simulink model "TP2_tanque_simulink_resp_impul"  (R2019b)
settings: Solver=VariableStepAuto  StartTime=0.0  StopTime=1500.0  RelTol=1e-3
values from neighbouring files (symbols this model uses):
  Ad = Hld_zoh.A    [TP2_rutina_minimos_cuadrados.m]    (also in tanque_simulink_param.m)
  alt_tank = 1    [TP2_rutina_minimos_cuadrados.m]    (also in tanque_simulink_param.m)
  ang = pi/3    (= 1.0471975512)    [TP2_rutina_minimos_cuadrados.m]    (also in tanque_simulink_param.m)
  Bd = Hld_zoh.B    [TP2_rutina_minimos_cuadrados.m]    (also in tanque_simulink_param.m)
  Cd = Hld_zoh.C    [TP2_rutina_minimos_cuadrados.m]    (also in tanque_simulink_param.m)
  d_p_apertura = 0.05    [TP2_rutina_minimos_cuadrados.m]    (also in tanque_simulink_param.m)
  Dd = Hld_zoh.D    [TP2_rutina_minimos_cuadrados.m]    (also in tanque_simulink_param.m)
  g = 9.8    [TP2_rutina_minimos_cuadrados.m]    (also in tanque_simulink_param.m)
  h0 = h0_array(i)    [TP2_rutina_minimos_cuadrados.m]    (also in tanque_simulink_param.m)
  p_apertura_lin = Q_ent/(pi*r_apertura^2) / (sqrt(2*g*h0))    [obtener_modelo_lineal.m]
  Q_ent = 0.0035    [TP2_rutina_minimos_cuadrados.m]    (also in tanque_simulink_param.m)
  r_apertura = 0.0254    [TP2_rutina_minimos_cuadrados.m]    (also in tanque_simulink_param.m)
  rad_menor = 0.05    [TP2_rutina_minimos_cuadrados.m]    (also in tanque_simulink_param.m)
  T0 = Ts    (= 1)    [TP2_rutina_minimos_cuadrados.m]    (also in tanque_simulink_param.m)
  Ts = 1    [TP2_rutina_minimos_cuadrados.m]    (also in tanque_simulink_param.m)
settings Model: Creator=Franco  LastModifiedBy=Franco

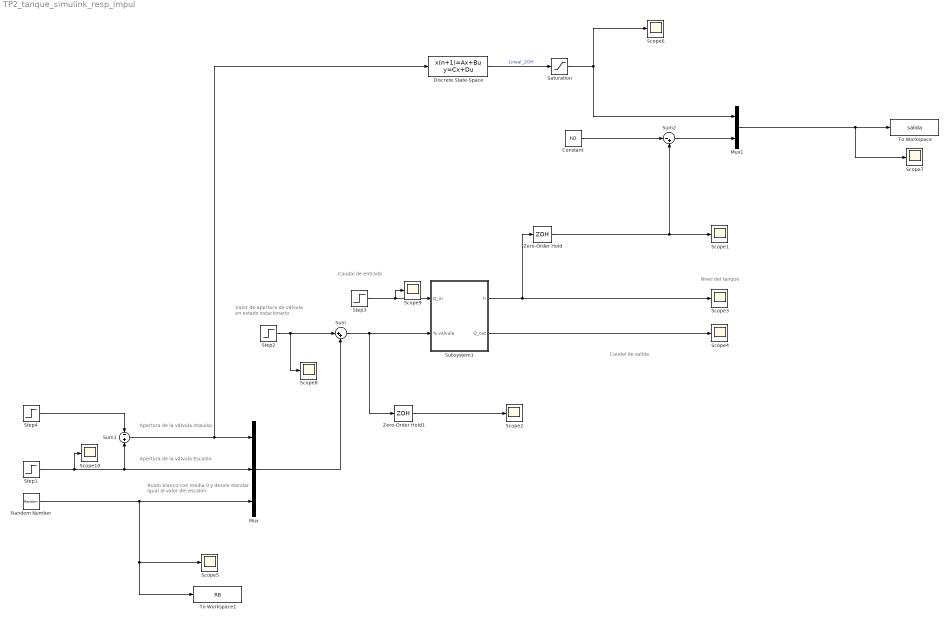
== system TP2_tanque_simulink_resp_impul ==
  note: Ruido blanco con media 0 y
      | desvío standar igual al valor del escalon
  note: Valor de apertura de válvula
      | en estado estacionario
  note: Apertura de la válvula
      | Escalón
  note: Caudal de salida
  note: Nivel del tanque
  note: Apertura de la válvula
      | Impulso
  note: Caudal de entrada
  Constant : Constant  Value=h0
  Discrete State-Space : DiscreteStateSpace  A=Ad  B=Bd  C=Cd  D=Dd  SampleTime=Ts
  Mux : Mux  Inputs=3
  Mux1 : Mux  Inputs=2
  Random Number : RandomNumber  Variance=(p_apertura_lin*d_p_apertura)^2  SampleTime=T0
  Saturation : Saturate  UpperLimit=alt_tank - h0  LowerLimit=-h0
  Scope{1..10} (10 alike) : Scope
  Step1 : Step  Time=T0  After=p_apertura_lin*d_p_apertura  SampleTime=0
  Step2 : Step  Time=T0/100  After=p_apertura_lin  SampleTime=0
  Step3 : Step  Time=T0/100  After=Q_ent  SampleTime=0
  Step4 : Step  Time=T0 + Ts  After=p_apertura_lin*d_p_apertura  SampleTime=0
  Subsystem1 : Subsystem
  Sum : Sum  Inputs=|++
  Sum1 : Sum  Inputs=-+
  Sum2 : Sum  Inputs=|-+
  To Workspace : ToWorkspace  VariableName=salida  SaveFormat=Timeseries  SampleTime=-1
      settings: Save2DSignal=2-D array (concatenate along first dimension)
  To Workspace1 : ToWorkspace  VariableName=RB  SaveFormat=Timeseries  SampleTime=-1
  Zero-Order Hold : ZeroOrderHold
  Zero-Order Hold1 : ZeroOrderHold
  wires:
  Step3/1 -> Scope9/1, Subsystem1/1(Q_in)
  Subsystem1/2(Q_out) -> Scope4/1
  Subsystem1/1(h) -> Zero-Order Hold/1, Scope3/1
  Zero-Order Hold/1 -> Sum2/2, Scope1/1
  Step1/1 -> Scope10/1, Mux/2, Sum1/2
  Zero-Order Hold1/1 -> Scope2/1
  Sum/1 -> Zero-Order Hold1/1, Subsystem1/2(" % válvula")
  Step2/1 -> Scope8/1, Sum/1
  Step4/1 -> Sum1/1
  Mux/1 -> Sum/2
  Random Number/1 -> To Workspace1/1, Scope5/1, Mux/3
  Discrete State-Space/1 -> Saturation/1  "Lineal_ZOH"
  Constant/1 -> Sum2/1
  Sum2/1 -> Mux1/2
  Sum1/1 -> Discrete State-Space/1, Mux/1
  Saturation/1 -> Scope6/1, Mux1/1
  Mux1/1 -> Scope7/1, To Workspace/1

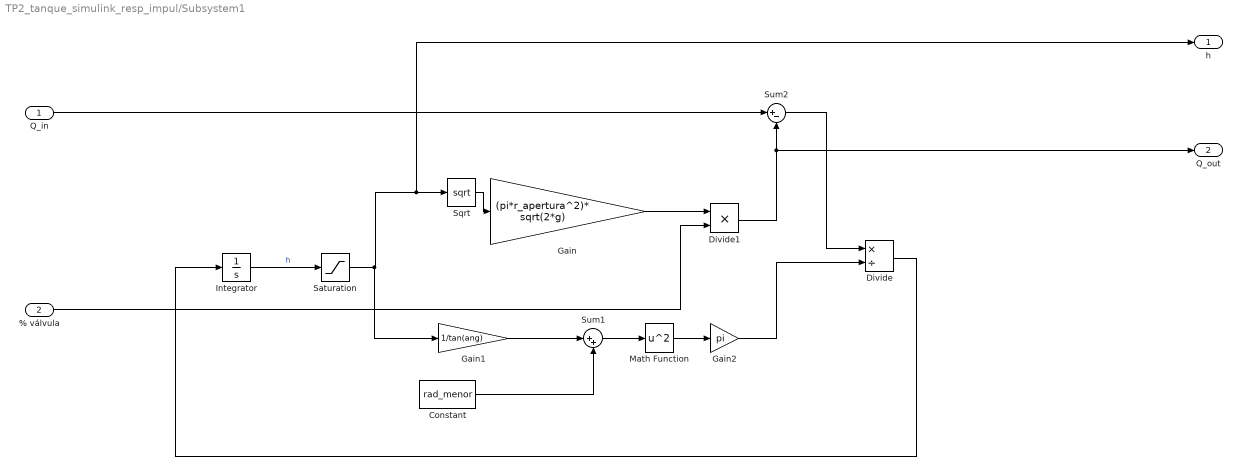
== system TP2_tanque_simulink_resp_impul/Subsystem1 ==
  Q_in : Inport
  " % válvula" : Inport  Port=2
  Constant : Constant  Value=rad_menor
  Divide : Product  Inputs=*/
  Divide1 : Product  Inputs=**
  Gain : Gain  Gain=(pi*r_apertura^2)* sqrt(2*g)
  Gain1 : Gain  Gain=1/tan(ang)
  Gain2 : Gain  Gain=pi
  Integrator : Integrator  InitialCondition=h0
  Math Function : Math  Operator=square  SignedPower=off  SaturateOnIntegerOverflow=on
  Saturation : Saturate  UpperLimit=1  LowerLimit=0
  Sqrt : Sqrt  SaturateOnIntegerOverflow=on
  Sum1 : Sum  Inputs=|++
  Sum2 : Sum  Inputs=|+-
  h : Outport
  Q_out : Outport  Port=2
  wires:
  Gain/1 -> Divide1/1
  Integrator/1 -> Saturation/1  "h"
  Sqrt/1 -> Gain/1
  Sum2/1 -> Divide/1
  Math Function/1 -> Gain2/1
  Saturation/1 -> Gain1/1, h/1, Sqrt/1
  Gain1/1 -> Sum1/1
  Sum1/1 -> Math Function/1
  Divide/1 -> Integrator/1
  Gain2/1 -> Divide/2
  Q_in/1 -> Sum2/1
  Constant/1 -> Sum1/2
  " % válvula"/1 -> Divide1/2
  Divide1/1 -> Q_out/1, Sum2/2
